simulink model "DTU_Topology_Medium_Line"  (R2023b)
settings: Solver=ode4  StartTime=0.0  StopTime=stoptime  FixedStep=Ts  RelTol=1e-3
PreLoadFcn:
  | Ts=1e-4;run('Grid_Parameters_3ph.m');load('Data_3ph_Pars.mat');load('First_Busbar_Pars.mat');load('PV_Busbar_Pars.mat');load('V2G_Busbar_Pars.mat');run('line_parameters.m')
PostLoadFcn:
  | Ts=1e-4;run('Grid_Parameters_3ph.m');load('Data_3ph_Pars.mat');load('First_Busbar_Pars.mat');load('PV_Busbar_Pars.mat');load('V2G_Busbar_Pars.mat');run('line_parameters.m')
InitFcn:
  | Ts=1e-4;run('Grid_Parameters_3ph.m');load('Data_3ph_Pars.mat');load('First_Busbar_Pars.mat');load('PV_Busbar_Pars.mat');load('V2G_Busbar_Pars.mat');run('line_parameters.m')
StartFcn:
  | Ts=1e-4;run('Grid_Parameters_3ph.m');load('Data_3ph_Pars.mat');load('First_Busbar_Pars.mat');load('PV_Busbar_Pars.mat');load('V2G_Busbar_Pars.mat');run('line_parameters.m')
values from neighbouring files (symbols this model uses):
  datastart = 6100    [Grid_Parameters_3ph.m]
  datastop = 6300    [Grid_Parameters_3ph.m]
  fnom = 50    [Grid_Parameters_3ph.m]    (also in line_parameters.m)
  line_param = struct()    [line_parameters.m]
  t_factor = 1/acceleration    (= 1)    [Grid_Parameters_3ph.m]
  timestep_meas_data = 1    [Grid_Parameters_3ph.m]
  Vnom = 400    [Grid_Parameters_3ph.m]
undefined symbols (not defined in the file or in its folder): another_event_name, Data_3ph_Pars, j, my_event_name, Newton, PV_Busbar_Pars, Raphson, V2G_Busbar_Pars
libraries: spsSeriesRLCBranchLib x57, spsGroundLib x30, spsThreePhaseVIMeasurementLib x17, spsControlledCurrentSourceLib x9, spsThreePhaseSineGeneratorLib x9, spsMeanLib x7, spsMutualInductanceLib x4, rtlab x2, spsThreePhaseSourceLib x1, sps_lib x1
(part 1 of 2)
Description:
  | Model of a simple control system for use iin training.
settings Model: VariantFading=off  Creator=Alex  LastModifiedBy=obus
settings SolverCC: AlgebraicLoopSolver=TrustRegion  AutoInsertRateTranBlk=on
settings DataIOCC: LimitDataPoints=on  SaveFormat=Array  SignalLoggingSaveFormat=ModelDataLogs  SaveOutput=off  SaveTime=off  ReturnWorkspaceOutputs=off  SignalLoggingName=sigsOut
settings OptimizationCC: BlockReduction=off  BooleanDataType=off  OptimizeBlockIOStorage=off  BufferReuse=off  GlobalBufferReuse=off  ExpressionFolding=off  LocalBlockOutputs=off  InitFltsAndDblsToZero=on  LifeSpan=inf  OptimizeDataStoreBuffers=off  BusAssignmentInplaceUpdate=off
settings DebuggingCC: SaveWithParameterizedLinksMsg=none  UnderspecifiedInitializationDetection=Classic  MergeDetectMultiDrivingBlocksExec=none  SignalResolutionControl=TryResolveAllWithWarning  MultiTaskDSMMsg=warning  MultiTaskCondExecSysMsg=none  FcnCallInpInsideContextMsg=warning  UnconnectedInputMsg=warning  UnconnectedOutputMsg=warning  UnconnectedLineMsg=warning  SFUnexpectedBacktrackingDiag=warning  SFNoUnconditionalDefaultTransitionDiag=warning  SFExecutionAtInitializationDiag=none  ArithmeticOperatorsInVariantConditions=warning
settings HardwareCC: ProdBitPerPointer=32  ProdBitPerSizeT=32  ProdBitPerPtrDiffT=32  ProdLargestAtomicFloat=None  ProdIntDivRoundTo=Undefined  ProdEndianess=Unspecified  ProdWordSize=32  ProdHWDeviceType=32-bit Generic  TargetUnknown=on
settings ModelReferenceCC: EnableRefExpFcnMdlSchedulingChecks=on  PropagateSignalLabelsOutOfModel=off
settings SFSimCC: SimUseLocalCustomCode=off  CustomCodeUndefinedFunction=UseInterfaceOnly
settings RTWCC: RTWUseLocalCustomCode=off  DLArmComputeVersion=19.05
settings CodeAppCC: StateflowObjectComments=on
settings GRTTargetCC: TargetFcnLib=ansi_tfl_tmw.mat  TargetLangStandard=C89/C90 (ANSI)  CombineOutputUpdateFcns=off  GRTInterface=on
settings ConfigComp: CovMetricSettings=dw  CovSaveCumulativeToWorkspaceVar=on  CovSaveSingleToWorkspaceVar=on  CovExternalEMLEnable=off

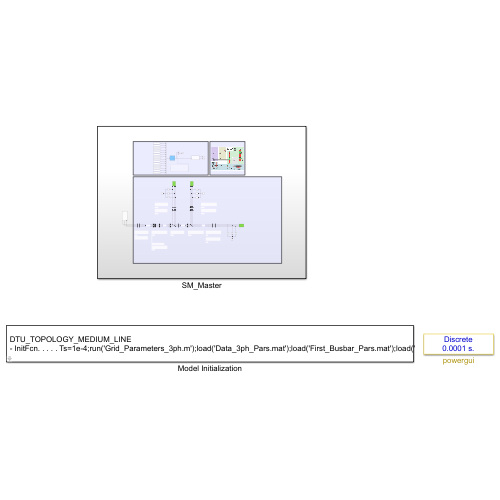
[thumbnail: Simulink's stored preview of the top-level diagram]
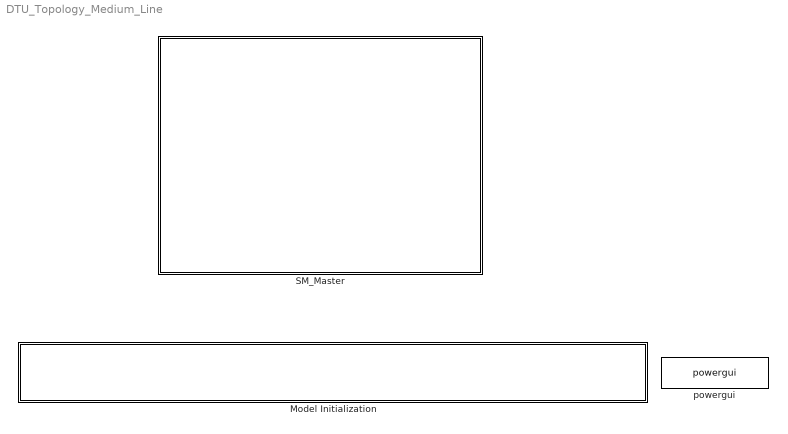
== system DTU_Topology_Medium_Line ==
  Model Initialization : Subsystem  mask(Model Functions){InitFcnX=Ts=1e-4;run('Grid_Parameters_3ph.m');load('Data_3ph_Pars.mat');load('First_Busbar_Pars.mat');load('PV_Busbar_Pars.mat');load('V2G_Busbar_Pars.mat');run('line_parameters.m'), prel=on, posl=on, inif=on, strf=on}
      mask prompts: InitFcnX "Initialisation"; prel "Preload Function"; posl "PostLoad Function"; inif "InitFcn"; strf "StartFcn"
      mask init:
      | currentBlock = gcb;
      | root = bdroot(currentBlock);
      | 
      | if ~strcmp(get_param(root,'BlockDiagramType'),'library')
      |     if prel==1
      |         set_param(root, 'PreLoadFcn', InitFcnX);
      |     else
      |         set_param(root, 'PreLoadFcn', '');
      |     end
      |     if inif==1
      |         set_param(root, 'InitFcn', InitFcnX);
      |     else
      |         set_param(root, 'InitFcn', '');
      |     end
      |     if strf==1
      |         set_param(root, 'StartFcn', InitFcnX);
      |     else
      |         set_param(root, 'StartFcn', '');
      |     end
      |     if posl==1
      |         set_param(root, 'PostLoadFcn', InitFcnX);
      |     else
      |         set_param(root, 'PostLoadFcn', '');
      |     end
      | end
      | 
      | pos = get_param(currentBlock, 'Position');
      | width = pos(3) - pos(1); height = pos(4) - pos(2);
      | txt = [ upper(root) '\n' '- InitFcn. . . . . '  get_param(root, 'InitFcn') ];
      settings: CopyFcn=set_param(gcb,'LinkStatus','none')
      mask Display: text(5, height*0.5, txt, 'horizontalAlignment', 'left', 'verticalAlignment', 'middle') ;
  SM_Master : Subsystem
  powergui : sps_lib/powergui  Priority=2  SimulationMode=Discrete  SampleTime=Ts  frequency=60  Iterations=50  frequencyindice=50  Pbase=100e6  ErrMax=1e-4  UnitsV=V  UnitsW=kW  buscounter=0  FunctionMessages=off  echomessages=off  EnableUseOfTLC=off  CurrentSourceSwitches=off  DisableSnubberDevices=off  DisableRonSwitches=off  DisableVfSwitches=off  DisplayEquations=off  AutomaticDiscreteSolvers=off  SolverType=Tustin  Interpol=off  ExternalGateDelay=off  methode=off  Ts=0  x0status=steady  SPID=off  SwTol=0  HookPort=off  NonlinearTolerance=0  nMaxIteration=15  ContinueOnMaxIteration=off  RestoreLinks=warning  ResistiveCurrentMeasurement=off  Frange=logspace(0,3,50)  Ylog=off  Xlog=off  ShowGrid=off  save=off  variable=ZData  structure=0  ZoomFFT=on  StartTime=0.0  cycles=1  DisplayStyle=1  fundamental=60  FreqAxis=off  MaxFrequency=1000  frequencyindicesteady=1  RmsSteady=2  display=off

== system DTU_Topology_Medium_Line/Model Initialization ==

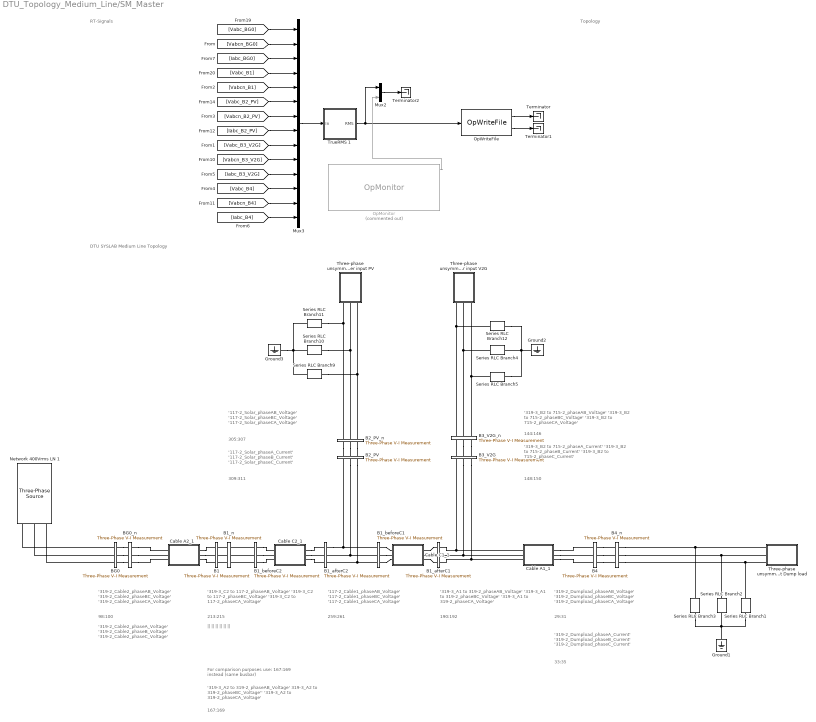
== system DTU_Topology_Medium_Line/SM_Master ==
  note: RT-Signals
  note: Topology
  note: DTU SYSLAB Medium Line Topology
  note: '319-3_C2 to 117-2_phaseAB_Voltage'
      | '319-3_C2 to 117-2_phaseBC_Voltage'
      | '319-3_C2 to 117-2_phaseCA_Voltage'
  note: '319-2_Dumpload_phaseAB_Voltage'
      | '319-2_Dumpload_phaseBC_Voltage'
      | '319-2_Dumpload_phaseCA_Voltage'
  note: '117-2_Cable1_phaseAB_Voltage'
      | '117-2_Cable1_phaseBC_Voltage'
      | '117-2_Cable1_phaseCA_Voltage'
  note: '319-2_Cable2_phaseAB_Voltage'
      | '319-2_Cable2_phaseBC_Voltage'
      | '319-2_Cable2_phaseCA_Voltage'
  note: '319-3_A1 to 319-2_phaseAB_Voltage'
      | '319-3_A1 to 319-2_phaseBC_Voltage'
      | '319-3_A1 to 319-2_phaseCA_Voltage'
  note: 98:100
  note: 213:215
  note: 259:261
  note: 190:192
  note: 29:31
  note: '319-3_B2 to 715-2_phaseA_Current'
      | '319-3_B2 to 715-2_phaseB_Current'
      | '319-3_B2 to 715-2_phaseC_Current'
  note: 148:150
  note: '117-2_Solar_phaseA_Current'
      | '117-2_Solar_phaseB_Current'
      | '117-2_Solar_phaseC_Current'
  note: 309:311
  note: '319-2_Dumpload_phaseA_Current'
      | '319-2_Dumpload_phaseB_Current'
      | '319-2_Dumpload_phaseC_Current'
  note: 33:35
  note: '117-2_Solar_phaseAB_Voltage'
      | '117-2_Solar_phaseBC_Voltage'
      | '117-2_Solar_phaseCA_Voltage'
  note: '319-3_B2 to 715-2_phaseAB_Voltage'
      | '319-3_B2 to 715-2_phaseBC_Voltage'
      | '319-3_B2 to 715-2_phaseCA_Voltage'
  note: 305:307
  note: 144:146
  note: 167:169
  note: '319-3_A2 to 319-2_phaseAB_Voltage'
      | 319-3_A2 to 319-2_phaseBC_Voltage''
      | '319-3_A2 to 319-2_phaseCA_Voltage'
  note: For comparison purposes use:
      | 167:169 instead (same busbar)
  note: ||
      | ||
      | ||
      | ||
      | ||
      | ||
  note: '319-2_Cable2_phaseA_Voltage'
      | '319-2_Cable2_phaseB_Voltage'
      | '319-2_Cable2_phaseC_Voltage'
  B1 : spsThreePhaseVIMeasurementLib/Three-Phase V-I Measurement  VoltageMeasurement=phase-to-phase  SetLabelV=on  LabelV=Vabc_B1  Vpu=off  VpuLL=off  CurrentMeasurement=no  SetLabelI=on  LabelI=Iabc_G2  Ipu=on  Pbase=900e6  Vbase=400  OutputType=Complex  PhasorSimulation=off  PSBequivalent=0
  B1_afterC1 : spsThreePhaseVIMeasurementLib/Three-Phase V-I Measurement  VoltageMeasurement=phase-to-ground  SetLabelV=on  LabelV=Vabcn_afterC1  Vpu=off  VpuLL=off  CurrentMeasurement=yes  SetLabelI=on  LabelI=Iabc_afterC1  Ipu=off  Pbase=900e6  Vbase=400  OutputType=Complex  PhasorSimulation=off  PSBequivalent=0
  B1_afterC2 : spsThreePhaseVIMeasurementLib/Three-Phase V-I Measurement  VoltageMeasurement=phase-to-ground  SetLabelV=on  LabelV=Vabcn_afterC2  Vpu=off  VpuLL=off  CurrentMeasurement=yes  SetLabelI=on  LabelI=Iabc_afterC2  Ipu=off  Pbase=900e6  Vbase=400  OutputType=Complex  PhasorSimulation=off  PSBequivalent=0
  B1_beforeC1 : spsThreePhaseVIMeasurementLib/Three-Phase V-I Measurement  VoltageMeasurement=phase-to-ground  SetLabelV=on  LabelV=Vabcn_beforeC1  Vpu=off  VpuLL=off  CurrentMeasurement=yes  SetLabelI=on  LabelI=Iabc_beforeC1  Ipu=off  Pbase=900e6  Vbase=400  OutputType=Complex  PhasorSimulation=off  PSBequivalent=0
  B1_beforeC2 : spsThreePhaseVIMeasurementLib/Three-Phase V-I Measurement  VoltageMeasurement=phase-to-ground  SetLabelV=on  LabelV=Vabcn_beforeC2  Vpu=off  VpuLL=off  CurrentMeasurement=yes  SetLabelI=on  LabelI=Iabc_beforeC2  Ipu=off  Pbase=900e6  Vbase=400  OutputType=Complex  PhasorSimulation=off  PSBequivalent=0
  B1_n : spsThreePhaseVIMeasurementLib/Three-Phase V-I Measurement  VoltageMeasurement=phase-to-ground  SetLabelV=on  LabelV=Vabcn_B1  Vpu=off  VpuLL=off  CurrentMeasurement=no  SetLabelI=on  LabelI=Iabc_before  Ipu=off  Pbase=900e6  Vbase=400  OutputType=Complex  PhasorSimulation=off  PSBequivalent=0
  B2_PV : spsThreePhaseVIMeasurementLib/Three-Phase V-I Measurement  VoltageMeasurement=phase-to-phase  SetLabelV=on  LabelV=Vabc_B2_PV  Vpu=off  VpuLL=off  CurrentMeasurement=yes  SetLabelI=on  LabelI=Iabc_B2_PV  Ipu=off  Pbase=900e6  Vbase=400  OutputType=Complex  PhasorSimulation=off  PSBequivalent=0
  B2_PV_n : spsThreePhaseVIMeasurementLib/Three-Phase V-I Measurement  VoltageMeasurement=phase-to-ground  SetLabelV=on  LabelV=Vabcn_B2_PV  Vpu=off  VpuLL=off  CurrentMeasurement=no  SetLabelI=on  LabelI=Iabc_B2_PV  Ipu=off  Pbase=900e6  Vbase=400  OutputType=Complex  PhasorSimulation=off  PSBequivalent=0
  B3_V2G : spsThreePhaseVIMeasurementLib/Three-Phase V-I Measurement  VoltageMeasurement=phase-to-phase  SetLabelV=on  LabelV=Vabc_B3_V2G  Vpu=off  VpuLL=off  CurrentMeasurement=yes  SetLabelI=on  LabelI=Iabc_B3_V2G  Ipu=off  Pbase=900e6  Vbase=400  OutputType=Complex  PhasorSimulation=off  PSBequivalent=0
  B3_V2G_n : spsThreePhaseVIMeasurementLib/Three-Phase V-I Measurement  VoltageMeasurement=phase-to-ground  SetLabelV=on  LabelV=Vabcn_B3_V2G  Vpu=off  VpuLL=off  CurrentMeasurement=no  SetLabelI=on  LabelI=Iabc_B3_V2G  Ipu=off  Pbase=900e6  Vbase=400  OutputType=Complex  PhasorSimulation=off  PSBequivalent=0
  B4 : spsThreePhaseVIMeasurementLib/Three-Phase V-I Measurement  VoltageMeasurement=phase-to-phase  SetLabelV=on  LabelV=Vabc_B4  Vpu=off  VpuLL=off  CurrentMeasurement=yes  SetLabelI=on  LabelI=Iabc_B4  Ipu=off  Pbase=900e6  Vbase=400  OutputType=Complex  PhasorSimulation=off  PSBequivalent=0
  B4_n : spsThreePhaseVIMeasurementLib/Three-Phase V-I Measurement  VoltageMeasurement=phase-to-ground  SetLabelV=on  LabelV=Vabcn_B4  Vpu=off  VpuLL=off  CurrentMeasurement=no  SetLabelI=on  LabelI=Iabc_B4  Ipu=off  Pbase=900e6  Vbase=400  OutputType=Complex  PhasorSimulation=off  PSBequivalent=0
  BG0 : spsThreePhaseVIMeasurementLib/Three-Phase V-I Measurement  VoltageMeasurement=phase-to-phase  SetLabelV=on  LabelV=Vabc_BG0  Vpu=off  VpuLL=off  CurrentMeasurement=yes  SetLabelI=on  LabelI=Iabc_BG0  Ipu=off  Pbase=900e6  Vbase=400  OutputType=Complex  PhasorSimulation=off  PSBequivalent=0
  BG0_n : spsThreePhaseVIMeasurementLib/Three-Phase V-I Measurement  VoltageMeasurement=phase-to-ground  SetLabelV=on  LabelV=Vabcn_BG0  Vpu=off  VpuLL=off  CurrentMeasurement=no  SetLabelI=on  LabelI=Iabc_BG0  Ipu=off  Pbase=900e6  Vbase=400  OutputType=Complex  PhasorSimulation=off  PSBequivalent=0
  Cable A1_1 : Subsystem  mask(ZHAW_Config){fNom=fnom, length=line_param.A1.length}
      mask prompts: fNom "Nominal frequency (Hz)"; length "Length (km)"
      mask Display:
      | patch([20 20 80 80], [0 20 20 0])
      | patch([0 0 20 20], [7 13 13 7])
      | patch([80 80 100 100], [7 13 13 7])
      | 
      | patch([20 20 80 80], [40 60 60 40])
      | patch([0 0 20 20], [47 53 53 47])
      | patch([80 80 100 100], [47 53 53 47])
      | 
      | patch([20 20 80 80], [80 100 100 80])
      | patch([0 0 20 20], [87 93 93 87])
      | patch([80 80 100 100], [87 93 93 87])
  Cable A2_1 : Subsystem  mask(ZHAW_Config){fNom=fnom, length=line_param.A2.length}
      mask prompts: fNom "Nominal frequency (Hz)"; length "Length (km)"
      mask Display:
      | patch([20 20 80 80], [0 20 20 0])
      | patch([0 0 20 20], [7 13 13 7])
      | patch([80 80 100 100], [7 13 13 7])
      | 
      | patch([20 20 80 80], [40 60 60 40])
      | patch([0 0 20 20], [47 53 53 47])
      | patch([80 80 100 100], [47 53 53 47])
      | 
      | patch([20 20 80 80], [80 100 100 80])
      | patch([0 0 20 20], [87 93 93 87])
      | patch([80 80 100 100], [87 93 93 87])
  Cable C1_1 : Subsystem  mask(ZHAW_Config){fNom=fnom, length=line_param.C1.length}
      mask prompts: fNom "Nominal frequency (Hz)"; length "Length (km)"
      mask Display:
      | patch([20 20 80 80], [0 20 20 0])
      | patch([0 0 20 20], [7 13 13 7])
      | patch([80 80 100 100], [7 13 13 7])
      | 
      | patch([20 20 80 80], [40 60 60 40])
      | patch([0 0 20 20], [47 53 53 47])
      | patch([80 80 100 100], [47 53 53 47])
      | 
      | patch([20 20 80 80], [80 100 100 80])
      | patch([0 0 20 20], [87 93 93 87])
      | patch([80 80 100 100], [87 93 93 87])
  Cable C2_1 : Subsystem  mask(ZHAW_Config){fNom=fnom, length=line_param.C2.length}
      mask prompts: fNom "Nominal frequency (Hz)"; length "Length (km)"
      mask Display:
      | patch([20 20 80 80], [0 20 20 0])
      | patch([0 0 20 20], [7 13 13 7])
      | patch([80 80 100 100], [7 13 13 7])
      | 
      | patch([20 20 80 80], [40 60 60 40])
      | patch([0 0 20 20], [47 53 53 47])
      | patch([80 80 100 100], [47 53 53 47])
      | 
      | patch([20 20 80 80], [80 100 100 80])
      | patch([0 0 20 20], [87 93 93 87])
      | patch([80 80 100 100], [87 93 93 87])
  Ground1 : spsGroundLib/Ground  LConnTagsString=a
  Ground2 : spsGroundLib/Ground  LConnTagsString=a
  Ground3 : spsGroundLib/Ground  LConnTagsString=a
  Mux2 : Mux  Inputs=2
  Mux3 : Mux  Inputs=3*ones(1,14)
  Network 400Vrms LN 1 : spsThreePhaseSourceLib/Three-Phase Source  InternalConnection=Yg  VoltagePhases=off  Voltage=400  PhaseAngle=0  Voltage_phases=[400 400 400]/sqrt(3)*1.00006  PhaseAngles_phases=[0 -120 +120]  Frequency=50  NonIdealSource=on  SpecifyImpedance=on  Resistance=400^2/10e6/10  Inductance=400^2/10e6/(2*pi*50)  ShortCircuitLevel=60e6  BaseVoltage=400  XRratio=1/0.1  BusType=swing  Pref=0  Qref=0  Prefabc=[10e3, 10e3, 10e3]  Qrefabc=[0, 0, 0]  Qmin=-Inf  Qmax=Inf
  OpMonitor : rtlab/Monitoring/OpMonitor  Commented=on  compute_time=on  real_step=on  idle_time=on  nb_overruns=on  user_time=off  user_name=my_event_name,another_event_name
      settings: SourceProductName=RT-LAB
  OpWriteFile : rtlab/DataLogging/OpWriteFile  Static_File=on  varname=med_line_case_4c  Filename=med_line_case_4c.mat  rtpath='./'  nrtpath='.\'  Acq_Group=26  file_size=[500e6]  write_offline=on  Sim_Mode=off  Nb_Samples=stoptime  Buffer_size=1000000
      settings: SourceProductName=RT-LAB  Decimation=10000
  Series RLC Branch{1..5,9..12} (9 alike) : spsSeriesRLCBranchLib/Series RLC Branch  LConnTagsString=__new0  RConnTagsString=__new0  BranchType=R  Resistance=1e12  Inductance=1e-3  SetiL0=off  InitialCurrent=0  Capacitance=1e-6  Setx0=off  InitialVoltage=0  Measurements=None
  Terminator : Terminator
  Terminator1 : Terminator
  Terminator2 : Terminator
  Three-phase unsymmetrical Dynamic Load Reactive Power input Dump load : Subsystem
  Three-phase unsymmetrical Dynamic Load Reactive Power input PV : Subsystem
  Three-phase unsymmetrical Dynamic Load Reactive Power input V2G : Subsystem
  TrueRMS 1 : Subsystem  AncestorBlock=powerlib_meascontrol/Measurements/RMS/TrueRMS
  wires:
  [Vabc_BG0] -> Mux3/1
  OpWriteFile/2 -> Terminator1/1
  OpWriteFile/1 -> Terminator/1
  Mux3/1 -> TrueRMS 1/1(In)
  TrueRMS 1/1(RMS) -> OpWriteFile/1, Mux2/1
  OpMonitor/1 -> Mux2/2
  Mux2/1 -> Terminator2/1
  [Vabc_B1] -> Mux3/4
  [Vabcn_B1] -> Mux3/5
  [Vabc_B2_PV] -> Mux3/6
  [Vabcn_B2_PV] -> Mux3/7
  [Iabc_B2_PV] -> Mux3/8
  [Vabc_B3_V2G] -> Mux3/9
  [Vabcn_B3_V2G] -> Mux3/10
  [Iabc_B3_V2G] -> Mux3/11
  [Iabc_B4] -> Mux3/14
  [Vabcn_BG0] -> Mux3/2
  [Iabc_BG0] -> Mux3/3
  [Vabcn_B4] -> Mux3/13
  [Vabc_B4] -> Mux3/12
  connections:
  Three-phase unsymmetrical Dynamic Load Reactive Power input Dump load/RConn1 -- B4_n/RConn1 -- Series RLC Branch3/LConn1
  Three-phase unsymmetrical Dynamic Load Reactive Power input Dump load/RConn3 -- B4_n/RConn3 -- Series RLC Branch1/LConn1
  Three-phase unsymmetrical Dynamic Load Reactive Power input Dump load/RConn2 -- B4_n/RConn2 -- Series RLC Branch2/LConn1
  Cable A1_1/RConn1 -- B4/LConn1
  Cable A1_1/RConn2 -- B4/LConn2
  Cable A1_1/RConn3 -- B4/LConn3
  Cable A1_1/LConn1 -- B3_V2G/LConn1 -- B1_afterC1/RConn1
  B3_V2G/LConn2 -- B1_afterC1/RConn2 -- Cable A1_1/LConn2
  B3_V2G/LConn3 -- B1_afterC1/RConn3 -- Cable A1_1/LConn3
  B1_afterC2/RConn1 -- B1_beforeC1/LConn1 -- B2_PV/LConn1
  B2_PV/LConn2 -- B1_beforeC1/LConn2 -- B1_afterC2/RConn2
  B2_PV/LConn3 -- B1_beforeC1/LConn3 -- B1_afterC2/RConn3
  Cable A2_1/RConn1 -- B1/LConn1
  Cable A2_1/RConn2 -- B1/LConn2
  Cable A2_1/RConn3 -- B1/LConn3
  Series RLC Branch10/LConn1 -- B2_PV_n/RConn2 -- Three-phase unsymmetrical Dynamic Load Reactive Power input PV/RConn2
  Series RLC Branch11/LConn1 -- B2_PV_n/RConn1 -- Three-phase unsymmetrical Dynamic Load Reactive Power input PV/RConn1
  Series RLC Branch9/LConn1 -- B2_PV_n/RConn3 -- Three-phase unsymmetrical Dynamic Load Reactive Power input PV/RConn3
  Series RLC Branch12/LConn1 -- B3_V2G_n/RConn1 -- Three-phase unsymmetrical Dynamic Load Reactive Power input V2G/RConn1
  Series RLC Branch4/LConn1 -- B3_V2G_n/RConn2 -- Three-phase unsymmetrical Dynamic Load Reactive Power input V2G/RConn2
  Series RLC Branch5/LConn1 -- B3_V2G_n/RConn3 -- Three-phase unsymmetrical Dynamic Load Reactive Power input V2G/RConn3
  Series RLC Branch5/RConn1 -- Ground2/LConn1 -- Series RLC Branch12/RConn1 -- Series RLC Branch4/RConn1
  Series RLC Branch3/RConn1 -- Ground1/LConn1 -- Series RLC Branch1/RConn1 -- Series RLC Branch2/RConn1
  Series RLC Branch9/RConn1 -- Ground3/LConn1 -- Series RLC Branch11/RConn1 -- Series RLC Branch10/RConn1
  BG0/RConn1 -- BG0_n/LConn1
  BG0/RConn2 -- BG0_n/LConn2
  BG0/RConn3 -- BG0_n/LConn3
  BG0_n/RConn1 -- Cable A2_1/LConn1
  BG0_n/RConn2 -- Cable A2_1/LConn2
  BG0_n/RConn3 -- Cable A2_1/LConn3
  B1_n/LConn1 -- B1/RConn1
  B1_n/LConn2 -- B1/RConn2
  B1_n/LConn3 -- B1/RConn3
  B2_PV_n/LConn1 -- B2_PV/RConn1
  B2_PV_n/LConn2 -- B2_PV/RConn2
  B2_PV_n/LConn3 -- B2_PV/RConn3
  B3_V2G/RConn1 -- B3_V2G_n/LConn1
  B3_V2G_n/LConn2 -- B3_V2G/RConn2
  B3_V2G_n/LConn3 -- B3_V2G/RConn3
  B4/RConn1 -- B4_n/LConn1
  B4/RConn2 -- B4_n/LConn2
  B4/RConn3 -- B4_n/LConn3
  BG0/LConn3 -- Network 400Vrms LN 1/RConn3
  BG0/LConn2 -- Network 400Vrms LN 1/RConn2
  BG0/LConn1 -- Network 400Vrms LN 1/RConn1
  Cable C2_1/RConn1 -- B1_afterC2/LConn1
  Cable C2_1/RConn2 -- B1_afterC2/LConn2
  Cable C2_1/RConn3 -- B1_afterC2/LConn3
  B1_beforeC2/LConn1 -- B1_n/RConn1
  B1_beforeC2/LConn2 -- B1_n/RConn2
  B1_beforeC2/LConn3 -- B1_n/RConn3
  B1_beforeC2/RConn2 -- Cable C2_1/LConn2
  B1_beforeC2/RConn1 -- Cable C2_1/LConn1
  B1_beforeC2/RConn3 -- Cable C2_1/LConn3
  B1_beforeC1/RConn1 -- Cable C1_1/LConn1
  B1_beforeC1/RConn2 -- Cable C1_1/LConn2
  B1_beforeC1/RConn3 -- Cable C1_1/LConn3
  Cable C1_1/RConn1 -- B1_afterC1/LConn1
  B1_afterC1/LConn2 -- Cable C1_1/RConn2
  Cable C1_1/RConn3 -- B1_afterC1/LConn3

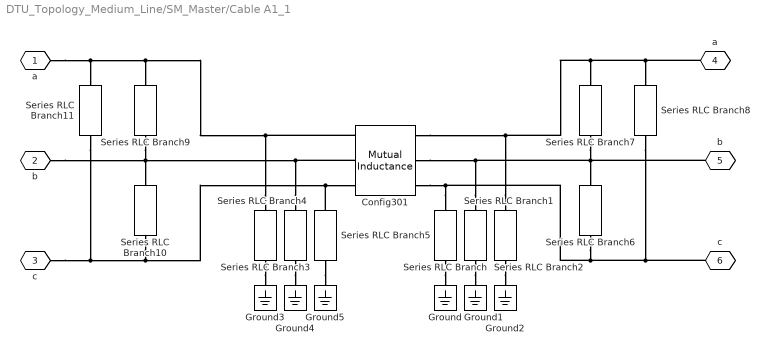
== system DTU_Topology_Medium_Line/SM_Master/Cable A1_1 ==
  Config301 : spsMutualInductanceLib/Mutual Inductance  LConnTagsString=a|b|c  RConnTagsString=A|B|C  TypeOfMutual=Generalized mutual inductance  NumberOfWindings=3  SelfImpedance1=[1.1 1.1e-03]  SelfImpedance2=[ 1.1 1.1e-03]  ThreeWindings=on  SelfImpedance3=[ 1.1 1.1e-03]  MutualImpedance=[1.0 1.0e-03]  InductanceMatrix=[line_param.A1.Ls line_param.A1.Lm line_param.A1.Lm ; line_param.A1.Lm line_param.A1.Ls line_param.A1.Lm ; line_param.A1.Lm line_param.A1.Lm line_param.A1.Ls]  ResistanceMatrix=[line_param.A1.Rs line_param.A1.Rm line_param.A1.Rm ; line_param.A1.Rm line_param.A1.Rs line_param.A1.Rm ; line_param.A1.Rm line_param.A1.Rm line_param.A1.Rs]  Measurements=None
      settings: LibrarySourceBlock=sps_lib/Passives/Mutual Inductance
  Ground{,1..5} (6 alike) : spsGroundLib/Ground  LConnTagsString=a
  Series RLC Branch{,1..5} (6 alike) : spsSeriesRLCBranchLib/Series RLC Branch  LConnTagsString=__new0  RConnTagsString=__new0  BranchType=C  Resistance=1  Inductance=1e-3  SetiL0=off  InitialCurrent=0  Capacitance=line_param.A1.Cg / 2  Setx0=off  InitialVoltage=0  Measurements=None
  Series RLC Branch{6..11} (6 alike) : spsSeriesRLCBranchLib/Series RLC Branch  LConnTagsString=__new0  RConnTagsString=__new0  BranchType=C  Resistance=1  Inductance=1e-3  SetiL0=off  InitialCurrent=0  Capacitance=line_param.A1.Cp / 2  Setx0=off  InitialVoltage=0  Measurements=None
  a : PMIOPort  Tag=PMCPort  Side=Left
  b : PMIOPort  Tag=PMCPort  Port=2  Side=Left
  c : PMIOPort  Tag=PMCPort  Port=3  Side=Left
  "a " : PMIOPort  Tag=PMCPort  Port=4  Side=Right
  "b " : PMIOPort  Tag=PMCPort  Port=5  Side=Right
  "c " : PMIOPort  Tag=PMCPort  Port=6  Side=Right
  connections:
  Series RLC Branch5/RConn1 -- Ground5/LConn1
  Series RLC Branch4/RConn1 -- Ground4/LConn1
  Series RLC Branch3/RConn1 -- Ground3/LConn1
  Series RLC Branch2/RConn1 -- Ground2/LConn1
  Series RLC Branch1/RConn1 -- Ground1/LConn1
  Series RLC Branch/RConn1 -- Ground/LConn1
  Series RLC Branch/LConn1 -- Config301/RConn3 -- Series RLC Branch8/RConn1 -- "c "/RConn1 -- Series RLC Branch6/RConn1
  Series RLC Branch1/LConn1 -- Config301/RConn2 -- Series RLC Branch7/RConn1 -- Series RLC Branch6/LConn1 -- "b "/RConn1
  Series RLC Branch2/LConn1 -- Config301/RConn1 -- Series RLC Branch8/LConn1 -- "a "/RConn1 -- Series RLC Branch7/LConn1
  Series RLC Branch5/LConn1 -- Config301/LConn3 -- Series RLC Branch11/RConn1 -- c/RConn1 -- Series RLC Branch10/RConn1
  Series RLC Branch4/LConn1 -- Config301/LConn2 -- Series RLC Branch10/LConn1 -- Series RLC Branch9/RConn1 -- b/RConn1
  Series RLC Branch3/LConn1 -- Config301/LConn1 -- Series RLC Branch11/LConn1 -- a/RConn1 -- Series RLC Branch9/LConn1

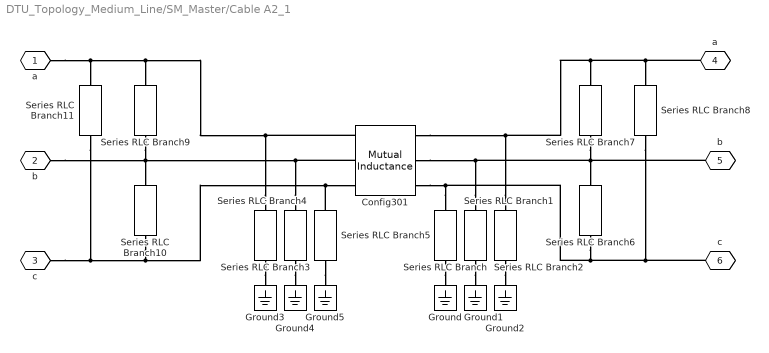
== system DTU_Topology_Medium_Line/SM_Master/Cable A2_1 ==
  Config301 : spsMutualInductanceLib/Mutual Inductance  LConnTagsString=a|b|c  RConnTagsString=A|B|C  TypeOfMutual=Generalized mutual inductance  NumberOfWindings=3  SelfImpedance1=[1.1 1.1e-03]  SelfImpedance2=[ 1.1 1.1e-03]  ThreeWindings=on  SelfImpedance3=[ 1.1 1.1e-03]  MutualImpedance=[1.0 1.0e-03]  InductanceMatrix=[line_param.A2.Ls line_param.A2.Lm line_param.A2.Lm ; line_param.A2.Lm line_param.A2.Ls line_param.A2.Lm ; line_param.A2.Lm line_param.A2.Lm line_param.A2.Ls]  ResistanceMatrix=[line_param.A2.Rs line_param.A2.Rm line_param.A2.Rm ; line_param.A2.Rm line_param.A2.Rs line_param.A2.Rm ; line_param.A2.Rm line_param.A2.Rm line_param.A2.Rs]  Measurements=None
      settings: LibrarySourceBlock=sps_lib/Passives/Mutual Inductance
  Ground{,1..5} (6 alike) : spsGroundLib/Ground  LConnTagsString=a
  Series RLC Branch{,1..5} (6 alike) : spsSeriesRLCBranchLib/Series RLC Branch  LConnTagsString=__new0  RConnTagsString=__new0  BranchType=C  Resistance=1  Inductance=1e-3  SetiL0=off  InitialCurrent=0  Capacitance=line_param.A2.Cg / 2  Setx0=off  InitialVoltage=0  Measurements=None
  Series RLC Branch{6..11} (6 alike) : spsSeriesRLCBranchLib/Series RLC Branch  LConnTagsString=__new0  RConnTagsString=__new0  BranchType=C  Resistance=1  Inductance=1e-3  SetiL0=off  InitialCurrent=0  Capacitance=line_param.A2.Cp / 2  Setx0=off  InitialVoltage=0  Measurements=None
  a : PMIOPort  Tag=PMCPort  Side=Left
  b : PMIOPort  Tag=PMCPort  Port=2  Side=Left
  c : PMIOPort  Tag=PMCPort  Port=3  Side=Left
  "a " : PMIOPort  Tag=PMCPort  Port=4  Side=Right
  "b " : PMIOPort  Tag=PMCPort  Port=5  Side=Right
  "c " : PMIOPort  Tag=PMCPort  Port=6  Side=Right
  connections:
  Series RLC Branch5/RConn1 -- Ground5/LConn1
  Series RLC Branch4/RConn1 -- Ground4/LConn1
  Series RLC Branch3/RConn1 -- Ground3/LConn1
  Series RLC Branch2/RConn1 -- Ground2/LConn1
  Series RLC Branch1/RConn1 -- Ground1/LConn1
  Series RLC Branch/RConn1 -- Ground/LConn1
  Series RLC Branch/LConn1 -- Config301/RConn3 -- Series RLC Branch8/RConn1 -- "c "/RConn1 -- Series RLC Branch6/RConn1
  Series RLC Branch1/LConn1 -- Config301/RConn2 -- Series RLC Branch7/RConn1 -- Series RLC Branch6/LConn1 -- "b "/RConn1
  Series RLC Branch2/LConn1 -- Config301/RConn1 -- Series RLC Branch8/LConn1 -- "a "/RConn1 -- Series RLC Branch7/LConn1
  Series RLC Branch5/LConn1 -- Config301/LConn3 -- Series RLC Branch11/RConn1 -- c/RConn1 -- Series RLC Branch10/RConn1
  Series RLC Branch4/LConn1 -- Config301/LConn2 -- Series RLC Branch10/LConn1 -- Series RLC Branch9/RConn1 -- b/RConn1
  Series RLC Branch3/LConn1 -- Config301/LConn1 -- Series RLC Branch11/LConn1 -- a/RConn1 -- Series RLC Branch9/LConn1

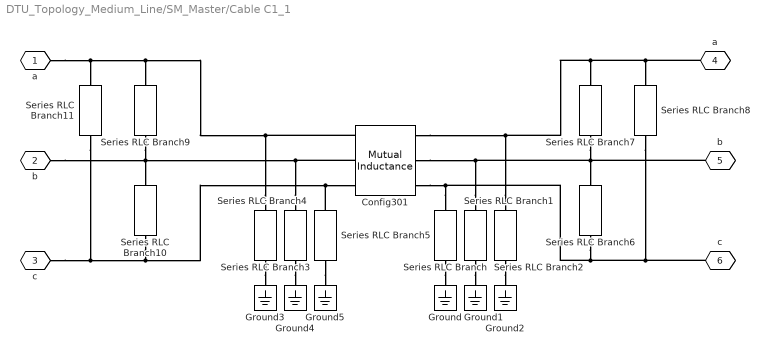
== system DTU_Topology_Medium_Line/SM_Master/Cable C1_1 ==
  Config301 : spsMutualInductanceLib/Mutual Inductance  LConnTagsString=a|b|c  RConnTagsString=A|B|C  TypeOfMutual=Generalized mutual inductance  NumberOfWindings=3  SelfImpedance1=[1.1 1.1e-03]  SelfImpedance2=[ 1.1 1.1e-03]  ThreeWindings=on  SelfImpedance3=[ 1.1 1.1e-03]  MutualImpedance=[1.0 1.0e-03]  InductanceMatrix=[line_param.C1.Ls line_param.C1.Lm line_param.C1.Lm ; line_param.C1.Lm line_param.C1.Ls line_param.C1.Lm ; line_param.C1.Lm line_param.C1.Lm line_param.C1.Ls]  ResistanceMatrix=[line_param.C1.Rs line_param.C1.Rm line_param.C1.Rm ; line_param.C1.Rm line_param.C1.Rs line_param.C1.Rm ; line_param.C1.Rm line_param.C1.Rm line_param.C1.Rs]  Measurements=None
      settings: LibrarySourceBlock=sps_lib/Passives/Mutual Inductance
  Ground{,1..5} (6 alike) : spsGroundLib/Ground  LConnTagsString=a
  Series RLC Branch{,1..5} (6 alike) : spsSeriesRLCBranchLib/Series RLC Branch  LConnTagsString=__new0  RConnTagsString=__new0  BranchType=C  Resistance=1  Inductance=1e-3  SetiL0=off  InitialCurrent=0  Capacitance=line_param.C1.Cg / 2  Setx0=off  InitialVoltage=0  Measurements=None
  Series RLC Branch{6..11} (6 alike) : spsSeriesRLCBranchLib/Series RLC Branch  LConnTagsString=__new0  RConnTagsString=__new0  BranchType=C  Resistance=1  Inductance=1e-3  SetiL0=off  InitialCurrent=0  Capacitance=line_param.C1.Cp / 2  Setx0=off  InitialVoltage=0  Measurements=None
  a : PMIOPort  Tag=PMCPort  Side=Left
  b : PMIOPort  Tag=PMCPort  Port=2  Side=Left
  c : PMIOPort  Tag=PMCPort  Port=3  Side=Left
  "a " : PMIOPort  Tag=PMCPort  Port=4  Side=Right
  "b " : PMIOPort  Tag=PMCPort  Port=5  Side=Right
  "c " : PMIOPort  Tag=PMCPort  Port=6  Side=Right
  connections:
  Series RLC Branch5/RConn1 -- Ground5/LConn1
  Series RLC Branch4/RConn1 -- Ground4/LConn1
  Series RLC Branch3/RConn1 -- Ground3/LConn1
  Series RLC Branch2/RConn1 -- Ground2/LConn1
  Series RLC Branch1/RConn1 -- Ground1/LConn1
  Series RLC Branch/RConn1 -- Ground/LConn1
  Series RLC Branch/LConn1 -- Config301/RConn3 -- Series RLC Branch8/RConn1 -- "c "/RConn1 -- Series RLC Branch6/RConn1
  Series RLC Branch1/LConn1 -- Config301/RConn2 -- Series RLC Branch7/RConn1 -- Series RLC Branch6/LConn1 -- "b "/RConn1
  Series RLC Branch2/LConn1 -- Config301/RConn1 -- Series RLC Branch8/LConn1 -- "a "/RConn1 -- Series RLC Branch7/LConn1
  Series RLC Branch5/LConn1 -- Config301/LConn3 -- Series RLC Branch11/RConn1 -- c/RConn1 -- Series RLC Branch10/RConn1
  Series RLC Branch4/LConn1 -- Config301/LConn2 -- Series RLC Branch10/LConn1 -- Series RLC Branch9/RConn1 -- b/RConn1
  Series RLC Branch3/LConn1 -- Config301/LConn1 -- Series RLC Branch11/LConn1 -- a/RConn1 -- Series RLC Branch9/LConn1

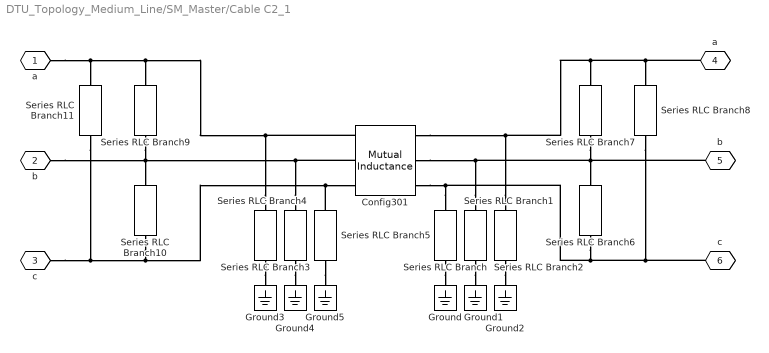
== system DTU_Topology_Medium_Line/SM_Master/Cable C2_1 ==
  Config301 : spsMutualInductanceLib/Mutual Inductance  LConnTagsString=a|b|c  RConnTagsString=A|B|C  TypeOfMutual=Generalized mutual inductance  NumberOfWindings=3  SelfImpedance1=[1.1 1.1e-03]  SelfImpedance2=[ 1.1 1.1e-03]  ThreeWindings=on  SelfImpedance3=[ 1.1 1.1e-03]  MutualImpedance=[1.0 1.0e-03]  InductanceMatrix=[line_param.C2.Ls line_param.C2.Lm line_param.C2.Lm ; line_param.C2.Lm line_param.C2.Ls line_param.C2.Lm ; line_param.C2.Lm line_param.C2.Lm line_param.C2.Ls]  ResistanceMatrix=[line_param.C2.Rs line_param.C2.Rm line_param.C2.Rm ; line_param.C2.Rm line_param.C2.Rs line_param.C2.Rm ; line_param.C2.Rm line_param.C2.Rm line_param.C2.Rs]  Measurements=None
      settings: LibrarySourceBlock=sps_lib/Passives/Mutual Inductance
  Ground{,1..5} (6 alike) : spsGroundLib/Ground  LConnTagsString=a
  Series RLC Branch{,1..5} (6 alike) : spsSeriesRLCBranchLib/Series RLC Branch  LConnTagsString=__new0  RConnTagsString=__new0  BranchType=C  Resistance=1  Inductance=1e-3  SetiL0=off  InitialCurrent=0  Capacitance=line_param.C2.Cg / 2  Setx0=off  InitialVoltage=0  Measurements=None
  Series RLC Branch{6..11} (6 alike) : spsSeriesRLCBranchLib/Series RLC Branch  LConnTagsString=__new0  RConnTagsString=__new0  BranchType=C  Resistance=1  Inductance=1e-3  SetiL0=off  InitialCurrent=0  Capacitance=line_param.C2.Cp / 2  Setx0=off  InitialVoltage=0  Measurements=None
  a : PMIOPort  Tag=PMCPort  Side=Left
  b : PMIOPort  Tag=PMCPort  Port=2  Side=Left
  c : PMIOPort  Tag=PMCPort  Port=3  Side=Left
  "a " : PMIOPort  Tag=PMCPort  Port=4  Side=Right
  "b " : PMIOPort  Tag=PMCPort  Port=5  Side=Right
  "c " : PMIOPort  Tag=PMCPort  Port=6  Side=Right
  connections:
  Series RLC Branch5/RConn1 -- Ground5/LConn1
  Series RLC Branch4/RConn1 -- Ground4/LConn1
  Series RLC Branch3/RConn1 -- Ground3/LConn1
  Series RLC Branch2/RConn1 -- Ground2/LConn1
  Series RLC Branch1/RConn1 -- Ground1/LConn1
  Series RLC Branch/RConn1 -- Ground/LConn1
  Series RLC Branch/LConn1 -- Config301/RConn3 -- Series RLC Branch8/RConn1 -- "c "/RConn1 -- Series RLC Branch6/RConn1
  Series RLC Branch1/LConn1 -- Config301/RConn2 -- Series RLC Branch7/RConn1 -- Series RLC Branch6/LConn1 -- "b "/RConn1
  Series RLC Branch2/LConn1 -- Config301/RConn1 -- Series RLC Branch8/LConn1 -- "a "/RConn1 -- Series RLC Branch7/LConn1
  Series RLC Branch5/LConn1 -- Config301/LConn3 -- Series RLC Branch11/RConn1 -- c/RConn1 -- Series RLC Branch10/RConn1
  Series RLC Branch4/LConn1 -- Config301/LConn2 -- Series RLC Branch10/LConn1 -- Series RLC Branch9/RConn1 -- b/RConn1
  Series RLC Branch3/LConn1 -- Config301/LConn1 -- Series RLC Branch11/LConn1 -- a/RConn1 -- Series RLC Branch9/LConn1

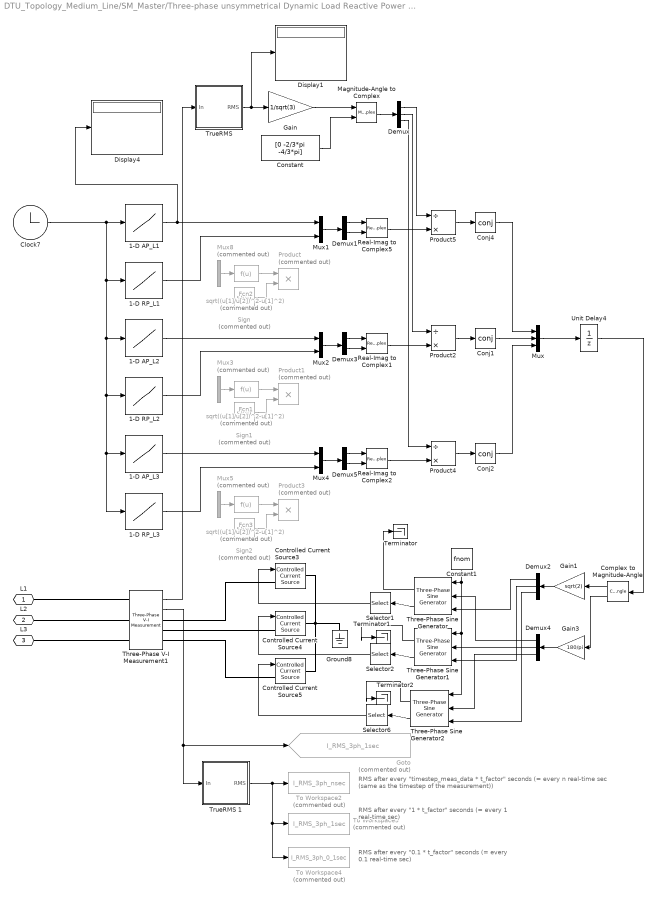
== system DTU_Topology_Medium_Line/SM_Master/Three-phase unsymmetrical Dynamic Load Reactive Power input Dump load ==
  note: RMS after every "1 * t_factor" seconds
      | (= every 1 real-time sec)
  note: RMS after every "0.1 * t_factor" seconds
      | (= every 0.1 real-time sec)
  note: RMS after every "timestep_meas_data * t_factor" seconds
      | (= every n real-time sec (same as the timestep of the measurement))
  1-D AP_L1 : Lookup_n-D  NumberOfTableDimensions=1  BreakpointsForDimension1=t_factor * [0:timestep_meas_data:(Data_3ph_Pars.Time(datastop)-Data_3ph_Pars.Time(datastart))]'  Table=Data_3ph_Pars.ActivePowerL1(datastart:datastop)  InterpMethod=Flat  InternalRulePriority=Speed  RndMeth=Simplest
  1-D AP_L2 : Lookup_n-D  NumberOfTableDimensions=1  BreakpointsForDimension1=t_factor * [0:timestep_meas_data:(Data_3ph_Pars.Time(datastop)-Data_3ph_Pars.Time(datastart))]'  Table=Data_3ph_Pars.ActivePowerL2(datastart:datastop)  InterpMethod=Flat  InternalRulePriority=Speed  RndMeth=Simplest
  1-D AP_L3 : Lookup_n-D  NumberOfTableDimensions=1  BreakpointsForDimension1=t_factor * [0:timestep_meas_data:(Data_3ph_Pars.Time(datastop)-Data_3ph_Pars.Time(datastart))]'  Table=Data_3ph_Pars.ActivePowerL3(datastart:datastop)  InterpMethod=Flat  InternalRulePriority=Speed  RndMeth=Simplest
  1-D RP_L1 : Lookup_n-D  NumberOfTableDimensions=1  BreakpointsForDimension1=t_factor * [0:timestep_meas_data:(Data_3ph_Pars.Time(datastop)-Data_3ph_Pars.Time(datastart))]'  Table=Data_3ph_Pars.ReactivePowerL1(datastart:datastop)  InterpMethod=Flat  InternalRulePriority=Speed  RndMeth=Simplest
  1-D RP_L2 : Lookup_n-D  NumberOfTableDimensions=1  BreakpointsForDimension1=t_factor * [0:timestep_meas_data:(Data_3ph_Pars.Time(datastop)-Data_3ph_Pars.Time(datastart))]'  Table=Data_3ph_Pars.ReactivePowerL2(datastart:datastop)  InterpMethod=Flat  InternalRulePriority=Speed  RndMeth=Simplest
  1-D RP_L3 : Lookup_n-D  NumberOfTableDimensions=1  BreakpointsForDimension1=t_factor * [0:timestep_meas_data:(Data_3ph_Pars.Time(datastop)-Data_3ph_Pars.Time(datastart))]'  Table=Data_3ph_Pars.ReactivePowerL3(datastart:datastop)  InterpMethod=Flat  InternalRulePriority=Speed  RndMeth=Simplest
  Clock7 : Clock
  Complex to Magnitude-Angle : ComplexToMagnitudeAngle
  Conj1 : Math  Operator=conj  SignedPower=on
  Conj2 : Math  Operator=conj  SignedPower=on
  Conj4 : Math  Operator=conj  SignedPower=on
  Constant : Constant  Value=[0 -2/3*pi -4/3*pi]
  Constant1 : Constant  Value=fnom
  Controlled Current Source3 : spsControlledCurrentSourceLib/Controlled Current Source  Initialize=on  Source_Type=AC  Amplitude=0  Phase=0  Frequency=50  Measurements=Current
  Controlled Current Source4 : spsControlledCurrentSourceLib/Controlled Current Source  Initialize=on  Source_Type=AC  Amplitude=0  Phase=0  Frequency=50  Measurements=Current
  Controlled Current Source5 : spsControlledCurrentSourceLib/Controlled Current Source  Initialize=on  Source_Type=AC  Amplitude=0  Phase=0  Frequency=50  Measurements=Current
  Demux : Demux  Outputs=3
  Demux1 : Demux  Outputs=2
      settings: DisplayOption=none
  Demux2 : Demux  Outputs=3
  Demux3 : Demux  Outputs=2
      settings: DisplayOption=none
  Demux4 : Demux  Outputs=3
  Demux5 : Demux  Outputs=2
      settings: DisplayOption=none
  Display1 : Display
  Display4 : Display
  Fcn1 : Fcn  Commented=on  Expr=sqrt((u[1]/u[2])^2-u[1]^2)
  Fcn2 : Fcn  Commented=on  Expr=sqrt((u[1]/u[2])^2-u[1]^2)
  Fcn3 : Fcn  Commented=on  Expr=sqrt((u[1]/u[2])^2-u[1]^2)
  Gain : Gain  Gain=1/sqrt(3)
  Gain1 : Gain  Gain=sqrt(2)
  Gain3 : Gain  Gain=180/pi
  Goto : Goto  Commented=on  GotoTag=I_RMS_3ph_1sec  TagVisibility=global
  Ground8 : spsGroundLib/Ground  LConnTagsString=a
  Magnitude-Angle to Complex : MagnitudeAngleToComplex
  Mux : Mux  Inputs=3
  Mux1 : Mux  Inputs=2
  Mux2 : Mux  Inputs=2
  Mux3 : Mux  Commented=on  Inputs=2
  Mux4 : Mux  Inputs=2
  Mux5 : Mux  Commented=on  Inputs=2
  Mux8 : Mux  Commented=on  Inputs=2
  Product : Product  Commented=on
  Product1 : Product  Commented=on
  Product2 : Product  Inputs=/*  InputSameDT=on  SaturateOnIntegerOverflow=on  OutDataTypeStr=Inherit: Same as first input
  Product3 : Product  Commented=on
  Product4 : Product  Inputs=/*  InputSameDT=on  SaturateOnIntegerOverflow=on  OutDataTypeStr=Inherit: Same as first input
  Product5 : Product  Inputs=/*  InputSameDT=on  SaturateOnIntegerOverflow=on  OutDataTypeStr=Inherit: Same as first input
  Real-Imag to Complex1 : RealImagToComplex
  Real-Imag to Complex2 : RealImagToComplex
  Real-Imag to Complex5 : RealImagToComplex
  Selector1 : Selector  InputPortWidth=3  IndexOptions=Index vector (dialog)  Indices=1  OutputSizes=1
  Selector2 : Selector  InputPortWidth=3  IndexOptions=Index vector (dialog)  Indices=1  OutputSizes=1
  Selector6 : Selector  InputPortWidth=3  IndexOptions=Index vector (dialog)  Indices=1  OutputSizes=1
  Sign : Signum  Commented=on
  Sign1 : Signum  Commented=on
  Sign2 : Signum  Commented=on
  Terminator : Terminator
  Terminator1 : Terminator
  Terminator2 : Terminator
  Three-Phase Sine Generator : spsThreePhaseSineGeneratorLib/Three-Phase Sine Generator  Ts=0
      settings: LibrarySourceBlock=|
      | sps_lib/Sources/Signal Generator Sources/Three-Phase
      | Sine Generator
  Three-Phase Sine Generator1 : spsThreePhaseSineGeneratorLib/Three-Phase Sine Generator  Ts=0
      settings: LibrarySourceBlock=|
      | sps_lib/Sources/Signal Generator Sources/Three-Phase
      | Sine Generator
  Three-Phase Sine Generator2 : spsThreePhaseSineGeneratorLib/Three-Phase Sine Generator  Ts=0
      settings: LibrarySourceBlock=|
      | sps_lib/Sources/Signal Generator Sources/Three-Phase
      | Sine Generator
  Three-Phase V-I Measurement1 : spsThreePhaseVIMeasurementLib/Three-Phase V-I Measurement  VoltageMeasurement=phase-to-phase  SetLabelV=off  LabelV=Vabc  Vpu=off  VpuLL=off  CurrentMeasurement=yes  SetLabelI=off  LabelI=Iabc  Ipu=off  Pbase=100e6  Vbase=Vnom*sqrt(3)  OutputType=Complex  PhasorSimulation=off  PSBequivalent=0
  To Workspace2 : ToWorkspace  Commented=on  VariableName=I_RMS_3ph_nsec  SampleTime=timestep_meas_data * t_factor
  To Workspace4 : ToWorkspace  Commented=on  VariableName=I_RMS_3ph_0_1sec  SampleTime=0.1 * t_factor
  To Workspace5 : ToWorkspace  Commented=on  VariableName=I_RMS_3ph_1sec  SampleTime=1 * t_factor
  "TrueRMS " : Subsystem  AncestorBlock=powerlib_meascontrol/Measurements/RMS/TrueRMS
  TrueRMS 1 : Subsystem  AncestorBlock=powerlib_meascontrol/Measurements/RMS/TrueRMS
  Unit Delay4 : UnitDelay  InitialCondition=0*exp(-j*0*pi/180)  SampleTime=Ts  HasFrameUpgradeWarning=on
  L1 : PMIOPort  Side=Right
  L2 : PMIOPort  Port=2  Side=Right
  L3 : PMIOPort  Port=3  Side=Right
  wires:
  1-D AP_L1/1 -> Display4/1, Mux1/1
  Product5/1 -> Conj4/1
  Fcn2/1 -> Product/1
  Three-Phase V-I Measurement1/2 -> Goto/1, TrueRMS 1/1(In)
  Mux1/1 -> Demux1/1
  Real-Imag to Complex5/1 -> Product5/2
  Clock7/1 -> 1-D RP_L1/1, 1-D RP_L2/1, 1-D AP_L3/1, 1-D RP_L3/1, 1-D AP_L2/1, 1-D AP_L1/1
  Sign/1 -> Product/2
  Mux8/1 -> Fcn2/1
  TrueRMS 1/1(RMS) -> To Workspace2/1, To Workspace5/1, To Workspace4/1
  Constant/1 -> Magnitude-Angle to Complex/2
  Demux/1 -> Product5/1
  Demux/2 -> Product2/1
  Demux/3 -> Product4/1
  Magnitude-Angle to Complex/1 -> Demux/1
  Gain/1 -> Magnitude-Angle to Complex/1
  Mux/1 -> Unit Delay4/1
  Complex to Magnitude-Angle/1 -> Gain1/1
  Three-Phase Sine Generator/1 -> Selector1/1
  Three-Phase Sine Generator1/1 -> Selector2/1
  Three-Phase Sine Generator2/1 -> Selector6/1
  Selector2/1 -> Controlled Current Source4/1
  Selector6/1 -> Controlled Current Source5/1
  Demux2/1 -> Three-Phase Sine Generator/1
  Demux2/2 -> Three-Phase Sine Generator1/1
  Demux2/3 -> Three-Phase Sine Generator2/1
  Conj4/1 -> Mux/1
  Conj1/1 -> Mux/2
  Conj2/1 -> Mux/3
  Constant1/1 -> Three-Phase Sine Generator/3, Three-Phase Sine Generator2/3, Three-Phase Sine Generator1/3
  Complex to Magnitude-Angle/2 -> Gain3/1
  Gain3/1 -> Demux4/1
  Selector1/1 -> Controlled Current Source3/1
  Demux4/1 -> Three-Phase Sine Generator/2
  Demux4/2 -> Three-Phase Sine Generator1/2
  Demux4/3 -> Three-Phase Sine Generator2/2
  Gain1/1 -> Demux2/1
  Demux1/1 -> Real-Imag to Complex5/1
  Demux1/2 -> Real-Imag to Complex5/2
  "TrueRMS "/1(RMS) -> Display1/1, Gain/1
  Three-Phase V-I Measurement1/1 -> "TrueRMS "/1(In)
  Unit Delay4/1 -> Complex to Magnitude-Angle/1
  Mux2/1 -> Demux3/1
  Demux3/2 -> Real-Imag to Complex1/2
  Real-Imag to Complex1/1 -> Product2/2
  Sign1/1 -> Product1/2
  Demux3/1 -> Real-Imag to Complex1/1
  Mux3/1 -> Fcn1/1
  1-D AP_L2/1 -> Mux2/1
  Product2/1 -> Conj1/1
  Fcn1/1 -> Product1/1
  Mux4/1 -> Demux5/1
  Demux5/2 -> Real-Imag to Complex2/2
  Real-Imag to Complex2/1 -> Product4/2
  Sign2/1 -> Product3/2
  Demux5/1 -> Real-Imag to Complex2/1
  Mux5/1 -> Fcn3/1
  1-D AP_L3/1 -> Mux4/1
  Product4/1 -> Conj2/1
  Fcn3/1 -> Product3/1
  1-D RP_L1/1 -> Mux1/2
  1-D RP_L2/1 -> Mux2/2
  1-D RP_L3/1 -> Mux4/2
  Three-Phase Sine Generator/2 -> Terminator/1
  Three-Phase Sine Generator1/2 -> Terminator1/1
  Three-Phase Sine Generator2/2 -> Terminator2/1
  connections:
  Three-Phase V-I Measurement1/RConn2 -- Controlled Current Source4/LConn1
  Three-Phase V-I Measurement1/RConn1 -- Controlled Current Source3/LConn1
  Three-Phase V-I Measurement1/RConn3 -- Controlled Current Source5/LConn1
  Controlled Current Source3/RConn1 -- Controlled Current Source4/RConn1 -- Ground8/LConn1 -- Controlled Current Source5/RConn1
  L1/RConn1 -- Three-Phase V-I Measurement1/LConn1
  Three-Phase V-I Measurement1/LConn2 -- L2/RConn1
  Three-Phase V-I Measurement1/LConn3 -- L3/RConn1
